simulink model "drone-tp-question5"  (R2025b)
settings: Solver=VariableStepAuto  StartTime=0.0  StopTime=10.0  RelTol=1e-3
values from neighbouring files (symbols this model uses):
  c = (b * sin(alpha)) / m    [drone-tp-observateur-commande.m]
  g = 9.81    [drone-tp-observateur-commande.m]
undefined symbols (not defined in the file or in its folder): A, B, C, D
settings Model: Creator=Etudiant  LastModifiedBy=Etudiant

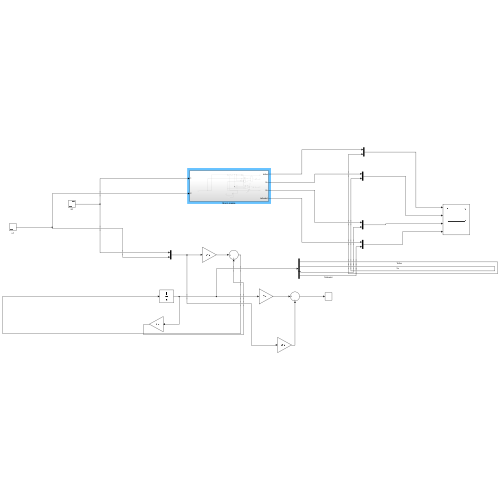
[thumbnail: Simulink's stored preview of the top-level diagram]
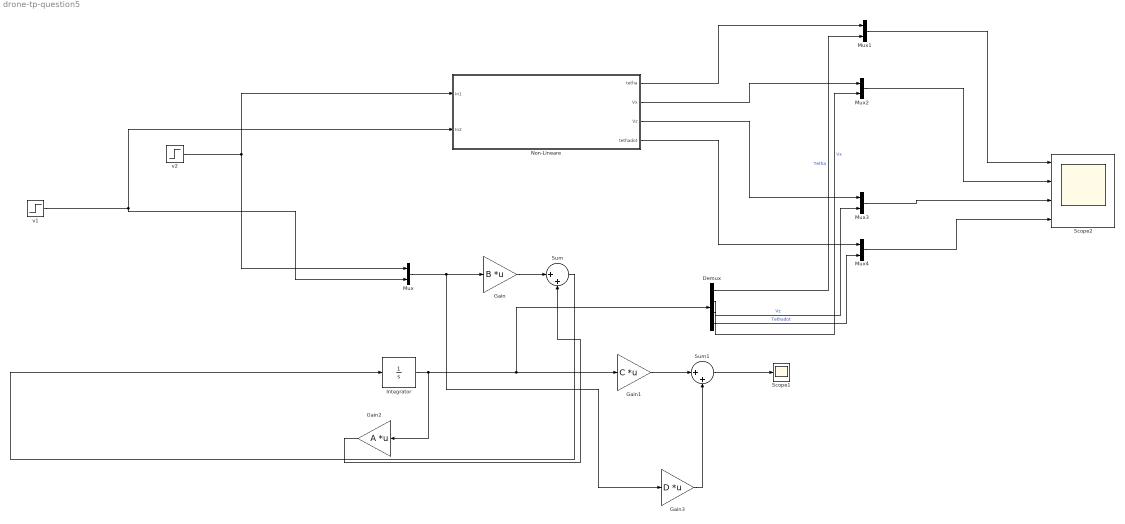
== system drone-tp-question5 ==
  Demux : Demux
  Gain : Gain  Gain=B  Multiplication=Matrix(K*u)
  Gain1 : Gain  Gain=C  Multiplication=Matrix(K*u)
  Gain2 : Gain  Gain=A  Multiplication=Matrix(K*u)
  Gain3 : Gain  Gain=D  Multiplication=Matrix(K*u)
  Integrator : Integrator
  Mux{,1..4} (5 alike) : Mux  Inputs=2
  Non-Lineare : Subsystem
  Scope1 : Scope
      settings: ActiveDisplayYMinimum=-1345.5813620155729  ActiveDisplayYMaximum=194.50904022395255  DataLoggingVariableName=ScopeData3
  Scope2 : Scope  NumInputPorts=4
      settings: ActiveDisplayYMinimum=-1340.5465354396995  ActiveDisplayYMaximum=149.14354052129929
  Sum : Sum  Inputs=|++
  Sum1 : Sum  Inputs=|++
  v1 : Step  SampleTime=0
  v2 : Step  After=0  SampleTime=0
  wires:
  Mux/1 -> Gain3/1, Gain/1
  Gain/1 -> Sum/1
  Sum/1 -> Integrator/1
  Gain2/1 -> Sum/2
  Gain1/1 -> Sum1/1
  Gain3/1 -> Sum1/2
  Sum1/1 -> Scope1/1
  Integrator/1 -> Demux/1, Gain1/1, Gain2/1
  Mux1/1 -> Scope2/1
  Mux2/1 -> Scope2/2
  Mux3/1 -> Scope2/3
  Mux4/1 -> Scope2/4
  Demux/1 -> Mux1/2  "Tetha"
  Demux/3 -> Mux3/2  "Vz"
  Demux/4 -> Mux4/2  "Tethadot"
  Demux/2 -> Mux2/2  "Vx"
  v1/1 -> Mux/2, Non-Lineare/2(In2)
  v2/1 -> Non-Lineare/1(In1), Mux/1
  Non-Lineare/1(tetha) -> Mux1/1
  Non-Lineare/2(Vx) -> Mux2/1
  Non-Lineare/3(Vz) -> Mux3/1
  Non-Lineare/4(tethadot) -> Mux4/1

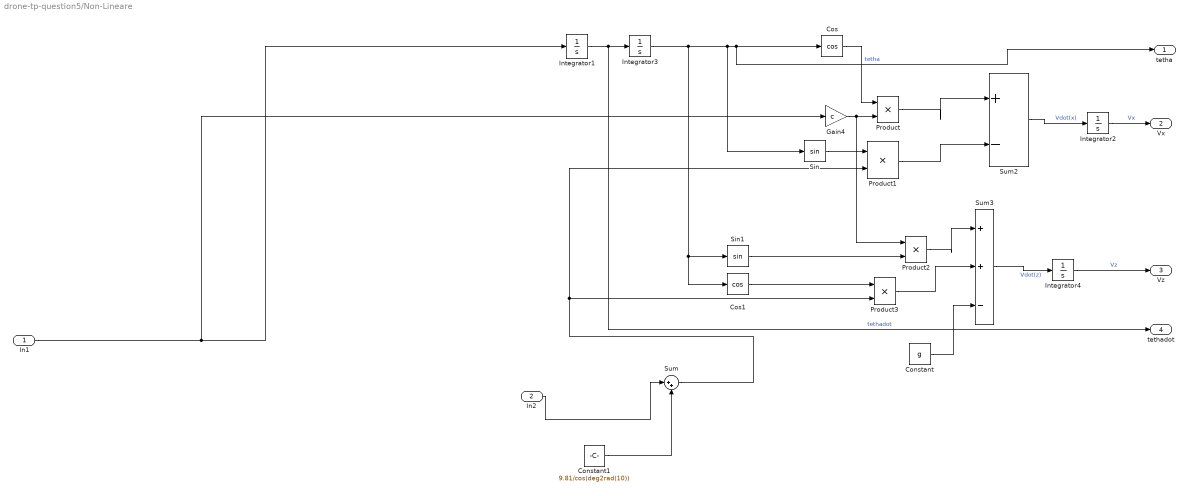
== system drone-tp-question5/Non-Lineare ==
  In1 : Inport
  In2 : Inport  Port=2
  Constant : Constant  Value=g
  Constant1 : Constant  Value=9.81/cos(deg2rad(10))
  Cos : Trigonometry  Operator=cos
  Cos1 : Trigonometry  Operator=cos
  Gain4 : Gain  Gain=c
  Integrator1 : Integrator
  Integrator2 : Integrator
  Integrator3 : Integrator  InitialCondition=deg2rad(10)
  Integrator4 : Integrator
  Product{,1..3} (4 alike) : Product
  Sin : Trigonometry
  Sin1 : Trigonometry
  Sum : Sum  Inputs=|++
  Sum2 : Sum  Inputs=|+-
  Sum3 : Sum  Inputs=|++-
  tetha : Outport
  Vx : Outport  Port=2
  Vz : Outport  Port=3
  tethadot : Outport  Port=4
  wires:
  Integrator2/1 -> Vx/1  "Vx"
  Sin1/1 -> Product2/2
  Cos1/1 -> Product3/1
  Integrator1/1 -> tethadot/1, Integrator3/1  "tethadot"
  Product1/1 -> Sum2/2
  Gain4/1 -> Product2/1, Product/2
  Sin/1 -> Product1/1
  Cos/1 -> Product/1
  Product2/1 -> Sum3/1
  In2/1 -> Sum/1
  In1/1 -> Integrator1/1, Gain4/1
  Product3/1 -> Sum3/2
  Product/1 -> Sum2/1
  Integrator3/1 -> Sin1/1, Cos1/1, tetha/1, Cos/1, Sin/1  "tetha"
  Constant/1 -> Sum3/3
  Sum2/1 -> Integrator2/1  "Vdot(x)"
  Sum3/1 -> Integrator4/1  "Vdot(z)"
  Integrator4/1 -> Vz/1  "Vz"
  Constant1/1 -> Sum/2
  Sum/1 -> Product1/2, Product3/2
